simulink model "Spacecraft_Model_HAVOC"  (R2022b)
settings: Solver=VariableStepAuto  StartTime=0.0  StopTime=300  RelTol=1e-3
model workspace (MAT data in the model file):
  R_0 = 80000
  Ts = 0.01
  mu = 398600.435507
undefined symbols (not defined in the file): As, c, q, SC
libraries: simulink x6, cstblocks x6, aerolibnav x6, matrix_library x4, sharedtransform x4, sharedTrackingLibrary x3, aerolibgravity2 x3, aerolibutil x2, sharedutil x1
settings Model: Creator=rohin  LastModifiedBy=rohin

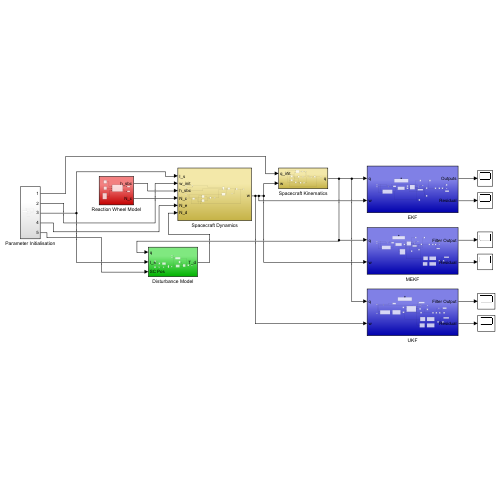
[thumbnail: Simulink's stored preview of the top-level diagram]
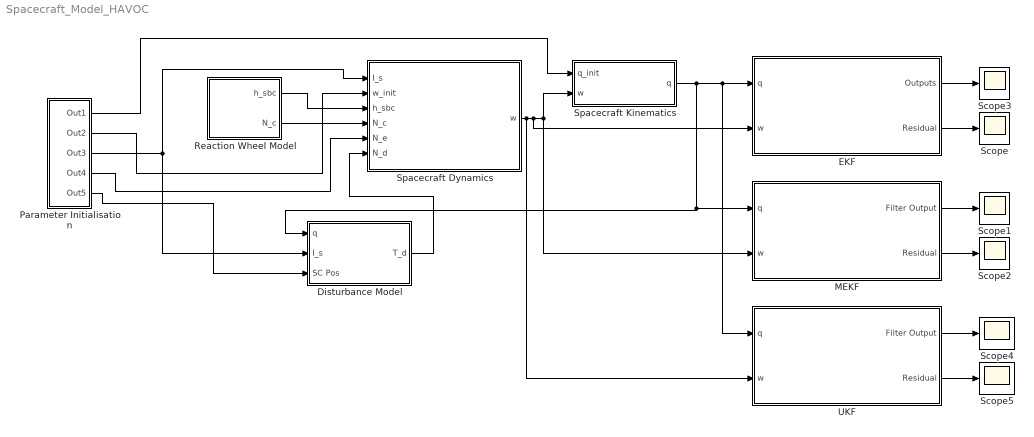
== system Spacecraft_Model_HAVOC ==
  Disturbance Model : Subsystem
  EKF : Subsystem
  MEKF : Subsystem
  Parameter Initialisation : Subsystem
  Reaction Wheel Model : Subsystem
  Scope{,1..5} (6 alike) : Scope
  Spacecraft Dynamics : Subsystem
  Spacecraft Kinematics : Subsystem
  UKF : Subsystem
  wires:
  Spacecraft Kinematics/1(q) -> MEKF/1(q), Disturbance Model/1(q), UKF/1(q), EKF/1(q)
  Spacecraft Dynamics/1(w) -> UKF/2(w), EKF/2(w), Spacecraft Kinematics/2(w), MEKF/2(w)
  EKF/1(Outputs) -> Scope3/1
  Reaction Wheel Model/1(h_sbc) -> Spacecraft Dynamics/3(h_sbc)
  Reaction Wheel Model/2(N_c) -> Spacecraft Dynamics/4(N_c)
  Disturbance Model/1(T_d) -> Spacecraft Dynamics/6(N_d)
  EKF/2(Residual) -> Scope/1
  MEKF/1(Filter Output) -> Scope1/1
  MEKF/2(Residual) -> Scope2/1
  UKF/1(Filter Output) -> Scope4/1
  UKF/2(Residual) -> Scope5/1
  Parameter Initialisation/3(Out3) -> Spacecraft Dynamics/1(I_s), Disturbance Model/2(I_s)
  Parameter Initialisation/1(Out1) -> Spacecraft Kinematics/1(q_init)
  Parameter Initialisation/2(Out2) -> Spacecraft Dynamics/2(w_init)
  Parameter Initialisation/4(Out4) -> Spacecraft Dynamics/5(N_e)
  Parameter Initialisation/5(Out5) -> Disturbance Model/3(SC Pos)

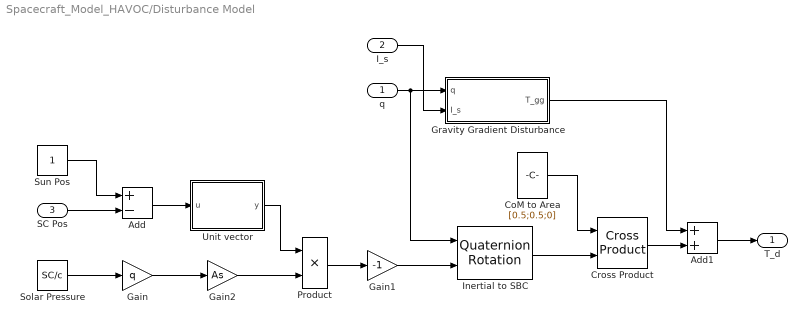
== system Spacecraft_Model_HAVOC/Disturbance Model ==
  q : Inport
  I_s : Inport  Port=2
  SC Pos : Inport  Port=3
  Add : Sum  Inputs=+-
  Add1 : Sum
  CoM to Area : Constant  Value=[0.5;0.5;0]  VectorParams1D=off
  Cross Product : matrix_library/Cross Product
  Gain : Gain  Gain=q
  Gain1 : Gain  Gain=-1
  Gain2 : Gain  Gain=As
  Gravity Gradient Disturbance : Subsystem
  Inertial to SBC : aerolibutil/Quaternion Rotation
  Product : Product
  Solar Pressure : Constant  Value=SC/c
  Sun Pos : Constant
  Unit vector : MATLAB Function  TreatAsAtomicUnit=on
  T_d : Outport
  wires:
  Sun Pos/1 -> Add/1
  Solar Pressure/1 -> Gain/1
  Unit vector/1(y) -> Product/1
  q/1 -> Gravity Gradient Disturbance/1(q), Inertial to SBC/1
  SC Pos/1 -> Add/2
  Add/1 -> Unit vector/1(u)
  I_s/1 -> Gravity Gradient Disturbance/2(I_s)
  Gain/1 -> Gain2/1
  Gain2/1 -> Product/2
  Product/1 -> Gain1/1
  Gain1/1 -> Inertial to SBC/2
  Gravity Gradient Disturbance/1(T_gg) -> Add1/1
  CoM to Area/1 -> Cross Product/1
  Inertial to SBC/1 -> Cross Product/2
  Cross Product/1 -> Add1/2
  Add1/1 -> T_d/1

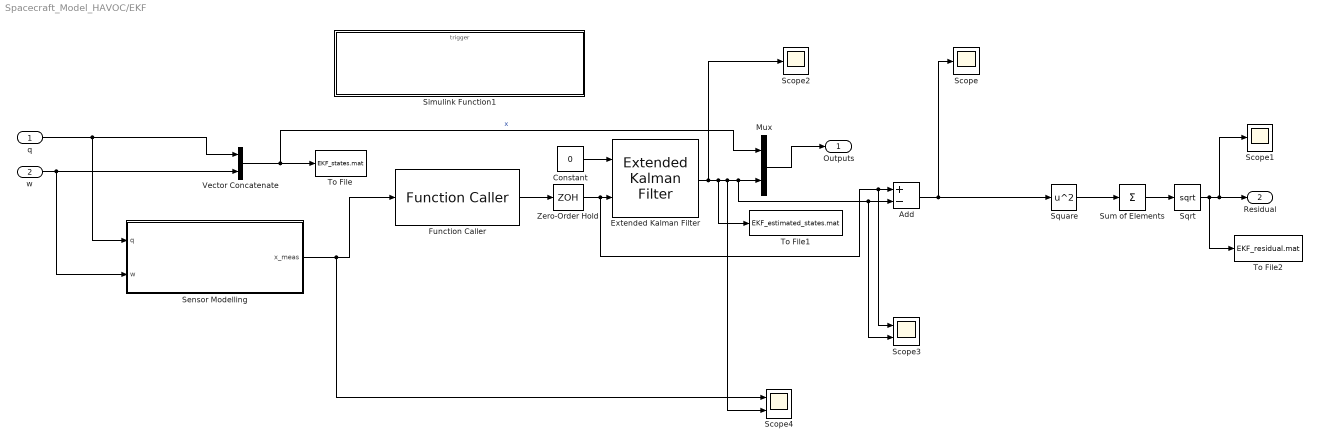
== system Spacecraft_Model_HAVOC/EKF ==
  q : Inport
  w : Inport  Port=2
  Add : Sum  Inputs=+-
  Constant : Constant  Value=0
  Extended Kalman Filter : sharedTrackingLibrary/Extended Kalman Filter  StateTransitionFcn=EKF_state_transition_func  HasStateTransitionJacobianFcn=off  HasAdditiveProcessNoise=Additive  ProcessNoise=0.05*diag([1,1,1,1,1,1,1])  HasTimeVaryingProcessNoise=off  HasStateTransitionFcnExtraArgument=1  InitialState=[1;0;0;0;0;0;0]  InitialStateCovariance=1  MeasurementFcn1=sensorMeasurementFcn  HasMeasurementJacobianFcn1=off  HasMeasurementEnablePort1=off  HasAdditiveMeasurementNoise1=Additive  MeasurementNoise1=0.1^2*diag([1,1,1,1,1,1,1])  HasTimeVaryingMeasurementNoise1=off  HasMeasurementFcnExtraArgument1=0  HasMeasurementWrapping1=off  MeasurementFcn2=myMeasurementFcn  HasMeasurementJacobianFcn2=off  HasMeasurementEnablePort2=off  HasAdditiveMeasurementNoise2=Additive  MeasurementNoise2=1  HasTimeVaryingMeasurementNoise2=off  HasMeasurementFcnExtraArgument2=0  HasMeasurementWrapping2=off  MeasurementFcn3=myMeasurementFcn  HasMeasurementJacobianFcn3=off  HasMeasurementEnablePort3=off  HasAdditiveMeasurementNoise3=Additive  MeasurementNoise3=1  HasTimeVaryingMeasurementNoise3=off  HasMeasurementFcnExtraArgument3=0  HasMeasurementWrapping3=off  MeasurementFcn4=myMeasurementFcn  HasMeasurementJacobianFcn4=off  HasMeasurementEnablePort4=off  HasAdditiveMeasurementNoise4=Additive  MeasurementNoise4=1  HasTimeVaryingMeasurementNoise4=off  HasMeasurementFcnExtraArgument4=0  HasMeasurementWrapping4=off  MeasurementFcn5=myMeasurementFcn  HasMeasurementJacobianFcn5=off  HasMeasurementEnablePort5=off  HasAdditiveMeasurementNoise5=Additive  MeasurementNoise5=1  HasTimeVaryingMeasurementNoise5=off  HasMeasurementFcnExtraArgument5=0  HasMeasurementWrapping5=off  EnableMultirate=off  StateTransitionFcnSampleTime=1  MeasurementFcn1SampleTime=1  MeasurementFcn2SampleTime=1  MeasurementFcn3SampleTime=1  MeasurementFcn4SampleTime=1  MeasurementFcn5SampleTime=1  UseCurrentEstimator=on  OutputStateCovariance=off  DataType=double  SampleTime=0.01  NumberOfMeasurements=1
  Function Caller : FunctionCaller  FunctionPrototype=y = sensorMeasurementFcn(x)  InputArgumentSpecifications=<Enter example>  OutputArgumentSpecifications=<Enter example>
  Mux : Mux  Inputs=2
  Scope : Scope
  Scope1 : Scope
  Scope2 : Scope
  Scope3 : Scope  NumInputPorts=2
  Scope4 : Scope  NumInputPorts=2
  "Sensor Modelling " : Subsystem
  Simulink Function1 : Subsystem  TreatAsAtomicUnit=on
  Sqrt : Sqrt
  Square : Math  Operator=square
  Sum of Elements : Sum  Inputs=+
  To File : ToFile  Filename=EKF_states.mat
  To File1 : ToFile  Filename=EKF_estimated_states.mat
  To File2 : ToFile  Filename=EKF_residual.mat
  Vector Concatenate : Concatenate
  Zero-Order Hold : ZeroOrderHold  SampleTime=0.01
  Outputs : Outport
  Residual : Outport  Port=2
  wires:
  Constant/1 -> Extended Kalman Filter/1
  w/1 -> "Sensor Modelling "/2(w), Vector Concatenate/2
  q/1 -> "Sensor Modelling "/1(q), Vector Concatenate/1
  Vector Concatenate/1 -> Mux/1, To File/1  "x"
  Function Caller/1 -> Zero-Order Hold/1
  Mux/1 -> Outputs/1
  Add/1 -> Square/1, Scope/1
  Sqrt/1 -> To File2/1, Scope1/1, Residual/1
  Square/1 -> Sum of Elements/1
  Sum of Elements/1 -> Sqrt/1
  "Sensor Modelling "/1(x_meas) -> Scope4/1, Function Caller/1
  Zero-Order Hold/1 -> Scope3/1, Add/1, Extended Kalman Filter/2
  Extended Kalman Filter/1 -> Scope2/1, Scope4/2, Add/2, Scope3/2, Mux/2, To File1/1

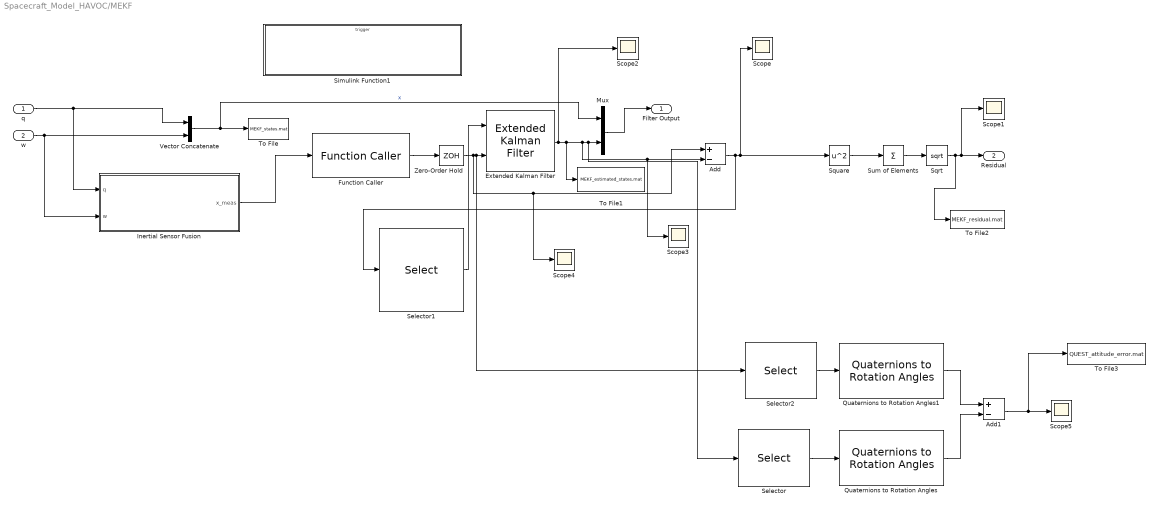
== system Spacecraft_Model_HAVOC/MEKF ==
  q : Inport
  w : Inport  Port=2
  Add : Sum  Inputs=+-
  Add1 : Sum  Inputs=+-
  Extended Kalman Filter : sharedTrackingLibrary/Extended Kalman Filter  StateTransitionFcn=MEKF_state_transition_func  HasStateTransitionJacobianFcn=off  HasAdditiveProcessNoise=Additive  ProcessNoise=0.5^2*diag([1,1,1,1,1,1,1])  HasTimeVaryingProcessNoise=off  HasStateTransitionFcnExtraArgument=1  InitialState=[1;0;0;0;0;0;0]  InitialStateCovariance=1  MeasurementFcn1=sensorMeasurementFcn  HasMeasurementJacobianFcn1=off  HasMeasurementEnablePort1=off  HasAdditiveMeasurementNoise1=Additive  MeasurementNoise1=0.01^2*diag([1,1,1,1,1,1,1])  HasTimeVaryingMeasurementNoise1=off  HasMeasurementFcnExtraArgument1=0  HasMeasurementWrapping1=off  MeasurementFcn2=myMeasurementFcn  HasMeasurementJacobianFcn2=off  HasMeasurementEnablePort2=off  HasAdditiveMeasurementNoise2=Additive  MeasurementNoise2=1  HasTimeVaryingMeasurementNoise2=off  HasMeasurementFcnExtraArgument2=0  HasMeasurementWrapping2=off  MeasurementFcn3=myMeasurementFcn  HasMeasurementJacobianFcn3=off  HasMeasurementEnablePort3=off  HasAdditiveMeasurementNoise3=Additive  MeasurementNoise3=1  HasTimeVaryingMeasurementNoise3=off  HasMeasurementFcnExtraArgument3=0  HasMeasurementWrapping3=off  MeasurementFcn4=myMeasurementFcn  HasMeasurementJacobianFcn4=off  HasMeasurementEnablePort4=off  HasAdditiveMeasurementNoise4=Additive  MeasurementNoise4=1  HasTimeVaryingMeasurementNoise4=off  HasMeasurementFcnExtraArgument4=0  HasMeasurementWrapping4=off  MeasurementFcn5=myMeasurementFcn  HasMeasurementJacobianFcn5=off  HasMeasurementEnablePort5=off  HasAdditiveMeasurementNoise5=Additive  MeasurementNoise5=1  HasTimeVaryingMeasurementNoise5=off  HasMeasurementFcnExtraArgument5=0  HasMeasurementWrapping5=off  EnableMultirate=off  StateTransitionFcnSampleTime=1  MeasurementFcn1SampleTime=1  MeasurementFcn2SampleTime=1  MeasurementFcn3SampleTime=1  MeasurementFcn4SampleTime=1  MeasurementFcn5SampleTime=1  UseCurrentEstimator=on  OutputStateCovariance=off  DataType=double  SampleTime=0.01  NumberOfMeasurements=1
  Function Caller : FunctionCaller  FunctionPrototype=y = sensorMeasurementFcn(x)  InputArgumentSpecifications=<Enter example>  OutputArgumentSpecifications=<Enter example>
  "Inertial Sensor Fusion " : Subsystem
  Mux : Mux  Inputs=2
  Quaternions to Rotation Angles : sharedtransform/Quaternions to Rotation Angles  rotationOrder=ZYX  aMode=aMode
  Quaternions to Rotation Angles1 : sharedtransform/Quaternions to Rotation Angles  rotationOrder=ZYX  aMode=aMode
  Scope{,1..5} (6 alike) : Scope
  Selector : Selector  InputPortWidth=7  IndexOptions=Index vector (dialog)  Indices=[1 2 3 4]  OutputSizes=1
  Selector1 : Selector  InputPortWidth=7  IndexOptions=Index vector (dialog)  Indices=[1 2 3 4]  OutputSizes=1
  Selector2 : Selector  InputPortWidth=7  IndexOptions=Index vector (dialog)  Indices=[1 2 3 4]  OutputSizes=1
  Simulink Function1 : Subsystem  TreatAsAtomicUnit=on
  Sqrt : Sqrt
  Square : Math  Operator=square
  Sum of Elements : Sum  Inputs=+
  To File : ToFile  Filename=MEKF_states.mat
  To File1 : ToFile  Filename=MEKF_estimated_states.mat
  To File2 : ToFile  Filename=MEKF_residual.mat
  To File3 : ToFile  Filename=QUEST_attitude_error.mat
  Vector Concatenate : Concatenate
  Zero-Order Hold : ZeroOrderHold  SampleTime=0.01
  Filter Output : Outport
  Residual : Outport  Port=2
  wires:
  Selector1/1 -> Extended Kalman Filter/1
  w/1 -> "Inertial Sensor Fusion "/2(w), Vector Concatenate/2
  q/1 -> "Inertial Sensor Fusion "/1(q), Vector Concatenate/1
  Vector Concatenate/1 -> Mux/1, To File/1  "x"
  Function Caller/1 -> Zero-Order Hold/1
  Mux/1 -> Filter Output/1
  "Inertial Sensor Fusion "/1(x_meas) -> Function Caller/1
  Sqrt/1 -> To File2/1, Scope1/1, Residual/1
  Square/1 -> Sum of Elements/1
  Sum of Elements/1 -> Sqrt/1
  Add/1 -> Selector1/1, Square/1, Scope/1
  Quaternions to Rotation Angles/1 -> Add1/2
  Quaternions to Rotation Angles1/1 -> Add1/1
  Add1/1 -> To File3/1, Scope5/1
  Zero-Order Hold/1 -> Scope4/1, Add/1, Selector2/1, Extended Kalman Filter/2
  Selector2/1 -> Quaternions to Rotation Angles1/1
  Selector/1 -> Quaternions to Rotation Angles/1
  Extended Kalman Filter/1 -> Scope2/1, Scope3/1, Add/2, Selector/1, Mux/2, To File1/1

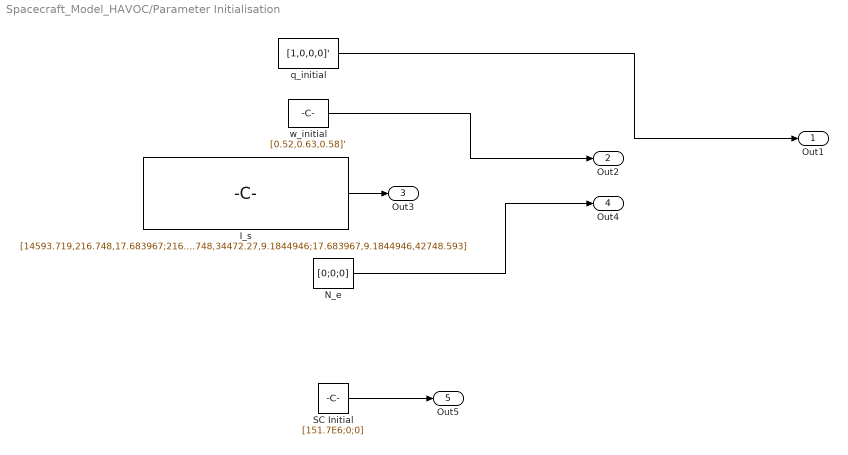
== system Spacecraft_Model_HAVOC/Parameter Initialisation ==
  I_s : Constant  Value=[14593.719,216.748,17.683967;216.748,34472.27,9.1844946;17.683967,9.1844946,42748.593]  VectorParams1D=off
  N_e : Constant  Value=[0;0;0]  VectorParams1D=off
  SC Initial : Constant  Value=[151.7E6;0;0]  VectorParams1D=off
  q_initial : Constant  Value=[1,0,0,0]'
  w_initial : Constant  Value=[0.52,0.63,0.58]'  VectorParams1D=off
  Out1 : Outport
  Out2 : Outport  Port=2
  Out3 : Outport  Port=3
  Out4 : Outport  Port=4
  Out5 : Outport  Port=5
  wires:
  I_s/1 -> Out3/1
  q_initial/1 -> Out1/1
  N_e/1 -> Out4/1
  w_initial/1 -> Out2/1
  SC Initial/1 -> Out5/1

== system Spacecraft_Model_HAVOC/Reaction Wheel Model ==
  N_d : Constant  Value=[5;0;0;0]  VectorParams1D=off
  Reaction Wheels : Subsystem
  beta : Constant  Value=45
  theta : Constant  Value=45
  h_sbc : Outport
  N_c : Outport  Port=2
  wires:
  Reaction Wheels/1(N_c) -> N_c/1
  beta/1 -> Reaction Wheels/2(beta)
  theta/1 -> Reaction Wheels/1(theta)
  N_d/1 -> Reaction Wheels/3(N_d)
  Reaction Wheels/2(h_sbc) -> h_sbc/1

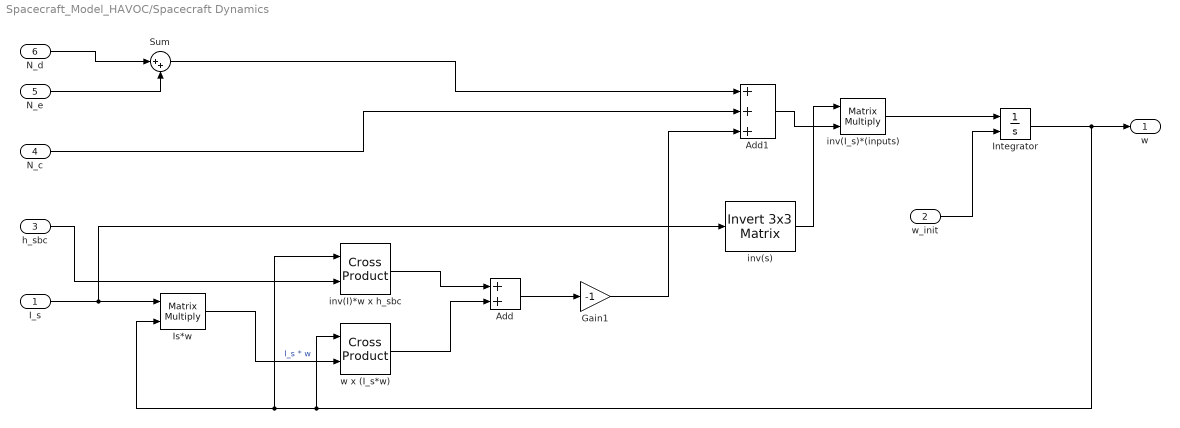
== system Spacecraft_Model_HAVOC/Spacecraft Dynamics ==
  I_s : Inport
  w_init : Inport  Port=2
  h_sbc : Inport  Port=3
  N_c : Inport  Port=4
  N_e : Inport  Port=5
  N_d : Inport  Port=6
  Add : Sum
  Add1 : Sum  Inputs=+++
  Gain1 : Gain  Gain=-1
  Integrator : Integrator  InitialConditionSource=external
  Is*w : Product  Multiplication=Matrix(*)
  Sum : Sum  Inputs=|++
  inv(I)*w x h_sbc : matrix_library/Cross Product
  inv(I_s)*(inputs) : Product  Multiplication=Matrix(*)
  inv(s) : aerolibutil/Invert  3x3 Matrix
  w x (I_s*w) : matrix_library/Cross Product
  w : Outport
  wires:
  w_init/1 -> Integrator/2
  Is*w/1 -> w x (I_s*w)/2  "I_s * w"
  N_c/1 -> Add1/2
  inv(I_s)*(inputs)/1 -> Integrator/1
  Integrator/1 -> w x (I_s*w)/1, inv(I)*w x h_sbc/1, Is*w/2, w/1
  I_s/1 -> inv(s)/1, Is*w/1
  inv(s)/1 -> inv(I_s)*(inputs)/1
  Add1/1 -> inv(I_s)*(inputs)/2
  h_sbc/1 -> inv(I)*w x h_sbc/2
  N_e/1 -> Sum/2
  N_d/1 -> Sum/1
  Sum/1 -> Add1/1
  w x (I_s*w)/1 -> Add/2
  inv(I)*w x h_sbc/1 -> Add/1
  Add/1 -> Gain1/1
  Gain1/1 -> Add1/3

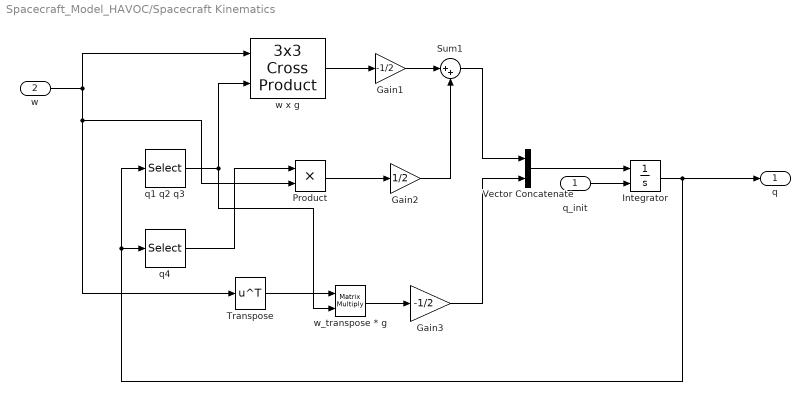
== system Spacecraft_Model_HAVOC/Spacecraft Kinematics ==
  q_init : Inport
  w : Inport  Port=2
  Gain1 : Gain  Gain=-1/2
  Gain2 : Gain  Gain=1/2
  Gain3 : Gain  Gain=-1/2
  Integrator : Integrator  InitialConditionSource=external
  Product : Product
  Sum1 : Sum  Inputs=|++
  Transpose : Math  Operator=transpose
  Vector Concatenate : Concatenate
  q1 q2 q3 : Selector  InputPortWidth=4  IndexOptions=Index vector (dialog)  Indices=[1 2 3]  OutputSizes=1
  q4 : Selector  InputPortWidth=4  IndexOptions=Index vector (dialog)  Indices=[4]  OutputSizes=1
  w x g : sharedutil/3x3 Cross Product  aMode=aMode
  w_transpose * g : Product  Multiplication=Matrix(*)
  q : Outport
  wires:
  Sum1/1 -> Vector Concatenate/1
  w_transpose * g/1 -> Gain3/1
  Gain1/1 -> Sum1/1
  Gain3/1 -> Vector Concatenate/2
  w x g/1 -> Gain1/1
  Gain2/1 -> Sum1/2
  w/1 -> Product/2, Transpose/1, w x g/1
  Transpose/1 -> w_transpose * g/1
  q1 q2 q3/1 -> w x g/2, w_transpose * g/2
  Vector Concatenate/1 -> Integrator/1
  q_init/1 -> Integrator/2
  Integrator/1 -> q/1, q1 q2 q3/1, q4/1
  q4/1 -> Product/1
  Product/1 -> Gain2/1

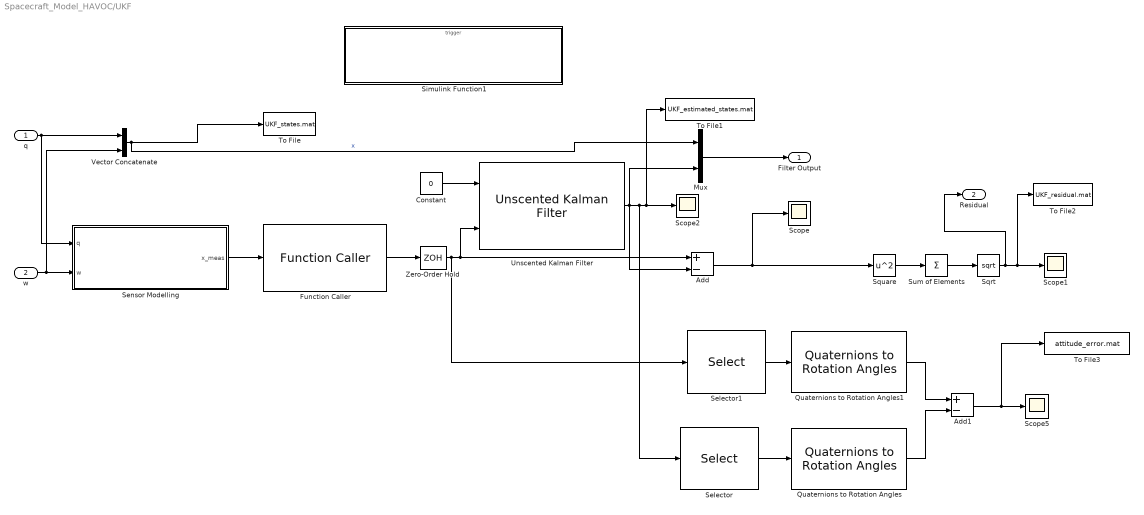
== system Spacecraft_Model_HAVOC/UKF ==
  q : Inport
  w : Inport  Port=2
  Add : Sum  Inputs=+-
  Add1 : Sum  Inputs=+-
  Constant : Constant  Value=0
  Function Caller : FunctionCaller  FunctionPrototype=y = UKF_sensorMeasurementFcn(x)  InputArgumentSpecifications=<Enter example>  OutputArgumentSpecifications=<Enter example>
  Mux : Mux  Inputs=2
  Quaternions to Rotation Angles : sharedtransform/Quaternions to Rotation Angles  rotationOrder=ZYX  aMode=aMode
  Quaternions to Rotation Angles1 : sharedtransform/Quaternions to Rotation Angles  rotationOrder=ZYX  aMode=aMode
  Scope{,1..2,5} (4 alike) : Scope
  Selector : Selector  InputPortWidth=7  IndexOptions=Index vector (dialog)  Indices=[1 2 3 4]  OutputSizes=1
  Selector1 : Selector  InputPortWidth=7  IndexOptions=Index vector (dialog)  Indices=[1 2 3 4]  OutputSizes=1
  "Sensor Modelling " : Subsystem
  Simulink Function1 : Subsystem  TreatAsAtomicUnit=on
  Sqrt : Sqrt
  Square : Math  Operator=square
  Sum of Elements : Sum  Inputs=+
  To File : ToFile  Filename=UKF_states.mat
  To File1 : ToFile  Filename=UKF_estimated_states.mat
  To File2 : ToFile  Filename=UKF_residual.mat
  To File3 : ToFile  Filename=attitude_error.mat
  Unscented Kalman Filter : sharedTrackingLibrary/Unscented Kalman Filter  StateTransitionFcn=UKF_state_transition_func  HasAdditiveProcessNoise=Additive  ProcessNoise=(0.1^2) * diag([0.01, 0.01, 0.01, 0.01, 0.01, 0.01, 0.01])  HasTimeVaryingProcessNoise=off  HasStateTransitionFcnExtraArgument=1  InitialState=[1;0;0;0;0;0;0]  InitialStateCovariance=0.01 * diag([0.01, 0.01, 0.01, 0.01, 0.01, 0.01, 0.01])  Alpha=1e-3  Beta=2  Kappa=0  MeasurementFcn1=UKF_sensorMeasurementFcn  HasMeasurementEnablePort1=off  HasAdditiveMeasurementNoise1=Additive  MeasurementNoise1=(0.001^2) * diag([0.01, 0.01, 0.01, 0.01, 0.01, 0.01, 0.01])  HasTimeVaryingMeasurementNoise1=off  HasMeasurementFcnExtraArgument1=0  HasMeasurementWrapping1=off  MeasurementFcn2=myMeasurementFcn  HasMeasurementEnablePort2=off  HasAdditiveMeasurementNoise2=Additive  MeasurementNoise2=1  HasTimeVaryingMeasurementNoise2=off  HasMeasurementFcnExtraArgument2=0  HasMeasurementWrapping2=off  MeasurementFcn3=myMeasurementFcn  HasMeasurementEnablePort3=off  HasAdditiveMeasurementNoise3=Additive  MeasurementNoise3=1  HasTimeVaryingMeasurementNoise3=off  HasMeasurementFcnExtraArgument3=0  HasMeasurementWrapping3=off  MeasurementFcn4=myMeasurementFcn  HasMeasurementEnablePort4=off  HasAdditiveMeasurementNoise4=Additive  MeasurementNoise4=1  HasTimeVaryingMeasurementNoise4=off  HasMeasurementFcnExtraArgument4=0  HasMeasurementWrapping4=off  MeasurementFcn5=myMeasurementFcn  HasMeasurementEnablePort5=off  HasAdditiveMeasurementNoise5=Additive  MeasurementNoise5=1  HasTimeVaryingMeasurementNoise5=off  HasMeasurementFcnExtraArgument5=0  HasMeasurementWrapping5=off  EnableMultirate=off  StateTransitionFcnSampleTime=1  MeasurementFcn1SampleTime=1  MeasurementFcn2SampleTime=1  MeasurementFcn3SampleTime=1  MeasurementFcn4SampleTime=1  MeasurementFcn5SampleTime=1  UseCurrentEstimator=on  OutputStateCovariance=off  DataType=double  SampleTime=0.01  NumberOfMeasurements=1
      settings: LibrarySourceBlock=cstblocks/State Estimation/Unscented Kalman Filter
  Vector Concatenate : Concatenate
  Zero-Order Hold : ZeroOrderHold  SampleTime=0.01
  Filter Output : Outport
  Residual : Outport  Port=2
  wires:
  q/1 -> "Sensor Modelling "/1(q), Vector Concatenate/1
  w/1 -> "Sensor Modelling "/2(w), Vector Concatenate/2
  Vector Concatenate/1 -> To File/1, Mux/1  "x"
  "Sensor Modelling "/1(x_meas) -> Function Caller/1
  Function Caller/1 -> Zero-Order Hold/1
  Constant/1 -> Unscented Kalman Filter/1
  Mux/1 -> Filter Output/1
  Add/1 -> Square/1, Scope/1
  Square/1 -> Sum of Elements/1
  Sum of Elements/1 -> Sqrt/1
  Sqrt/1 -> To File2/1, Scope1/1, Residual/1
  Quaternions to Rotation Angles/1 -> Add1/2
  Selector1/1 -> Quaternions to Rotation Angles1/1
  Quaternions to Rotation Angles1/1 -> Add1/1
  Unscented Kalman Filter/1 -> Selector/1, To File1/1, Scope2/1, Mux/2, Add/2
  Selector/1 -> Quaternions to Rotation Angles/1
  Zero-Order Hold/1 -> Selector1/1, Unscented Kalman Filter/2, Add/1
  Add1/1 -> To File3/1, Scope5/1

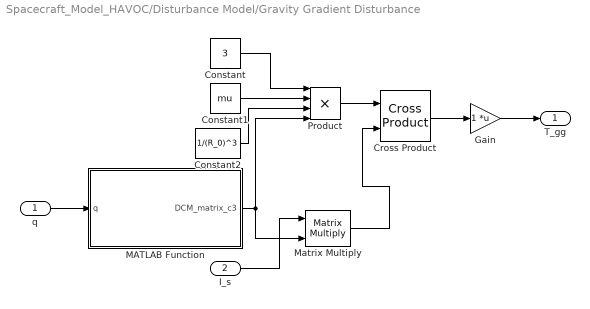
== system Spacecraft_Model_HAVOC/Disturbance Model/Gravity Gradient Disturbance ==
  q : Inport
  I_s : Inport  Port=2
  Constant : Constant  Value=3
  Constant1 : Constant  Value=mu
  Constant2 : Constant  Value=1/(R_0)^3
  Cross Product : matrix_library/Cross Product
  Gain : Gain  Multiplication=Matrix(K*u)
  MATLAB Function : MATLAB Function  TreatAsAtomicUnit=on
  Matrix Multiply : Product  Multiplication=Matrix(*)
  Product : Product  Inputs=4
  T_gg : Outport
  wires:
  q/1 -> MATLAB Function/1(q)
  Constant/1 -> Product/1
  Product/1 -> Cross Product/1
  MATLAB Function/1(DCM_matrix_c3) -> Matrix Multiply/2, Product/4
  Constant1/1 -> Product/2
  I_s/1 -> Matrix Multiply/1
  Matrix Multiply/1 -> Cross Product/2
  Constant2/1 -> Product/3
  Cross Product/1 -> Gain/1
  Gain/1 -> T_gg/1

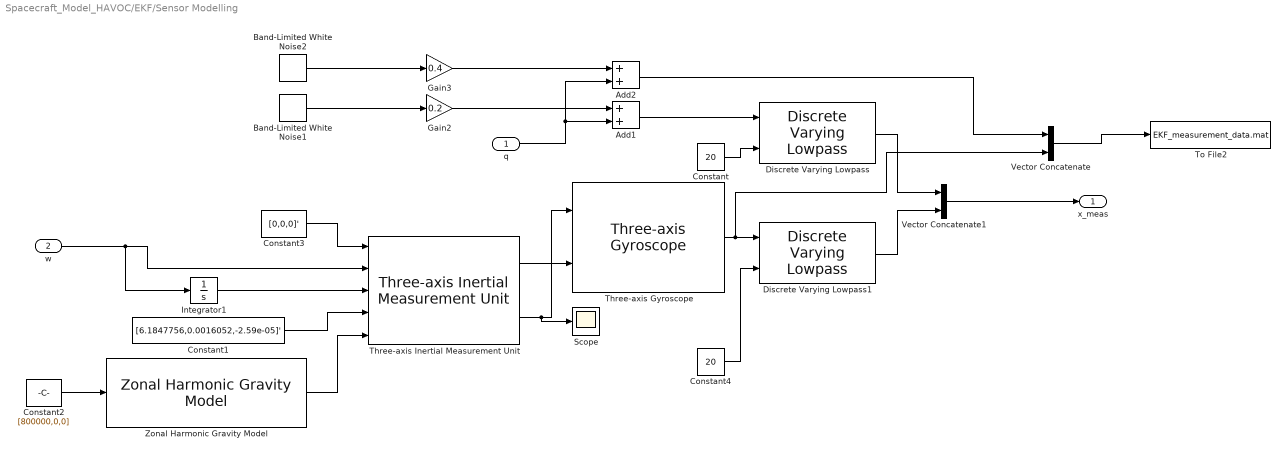
== system Spacecraft_Model_HAVOC/EKF/Sensor Modelling  ==
  q : Inport
  w : Inport  Port=2
  Add1 : Sum
  Add2 : Sum
  Band-Limited White Noise1 : simulink/Sources/Band-Limited White Noise  Cov=0.01  Ts=0.1  seed=[23341]
  Band-Limited White Noise2 : simulink/Sources/Band-Limited White Noise  Cov=0.01  Ts=0.1  seed=[23145]
  Constant : Constant  Value=20
  Constant1 : Constant  Value=[6.1847756,0.0016052,-2.59e-05]'
  Constant2 : Constant  Value=[800000,0,0]
  Constant3 : Constant  Value=[0,0,0]'
  Constant4 : Constant  Value=20
  Discrete Varying Lowpass : cstblocks/Linear Parameter Varying/Discrete Varying Lowpass  N=2  w0=0  Ts=0.01
  Discrete Varying Lowpass1 : cstblocks/Linear Parameter Varying/Discrete Varying Lowpass  N=2  w0=0  Ts=0.01
  Gain2 : Gain  Gain=0.2
  Gain3 : Gain  Gain=0.4
  Integrator1 : Integrator
  Scope : Scope
  Three-axis Gyroscope : aerolibnav/Three-axis Gyroscope  dtype_g=on  w_g=190  z_g=0.707  g_sf_cc=[1 0 0; 0 1 0; 0 0 1]  g_bias=0.0005*[1 1 1]  g_sen=[0 0 0]  g_Ts=0  g_rand=on  g_seeds=[23093 23094 23095]  g_pow=[0.0001 0.0001 0.0001]  g_sat="[-inf  -inf  -inf  inf inf inf]"
  Three-axis Inertial Measurement Unit : aerolibnav/Three-axis Inertial Measurement Unit  units=Metric (MKS)  imu=[0 0 0]  i_Ts=0  dtype_a=on  w_a=190  z_a=0.707  a_sf_cc=[1 0 0; 0 1 0; 0 0 1]  a_bias=[0 0 0]  a_sat="[-inf  -inf  -inf  inf inf inf]"  dtype_g=on  w_g=190  z_g=0.707  g_sf_cc=[1 0 0; 0 1 0; 0 0 1]  g_bias=[0 0 0]  g_sens=[0 0 0]  g_sat="[-inf  -inf  -inf  inf inf inf]"  i_rand=on  i_seeds=[23093 23094 23095 23096 23097 23098]  i_pow=[0.001 0.001 0.001 0.0001 0.0001 0.0001]
  To File2 : ToFile  Filename=EKF_measurement_data.mat
  Vector Concatenate : Concatenate
  Vector Concatenate1 : Concatenate
  Zonal Harmonic Gravity Model : aerolibgravity2/Zonal Harmonic Gravity Model  units=Metric (MKS)  degree=4  action=Warning  ptype=Earth  R=6378136.3  GM=398600441500000  jvalue=[1.0826269e-03 -2.5323000e-06 -1.6204000e-06]
  x_meas : Outport
  wires:
  Gain3/1 -> Add2/1
  Constant3/1 -> Three-axis Inertial Measurement Unit/1
  w/1 -> Three-axis Inertial Measurement Unit/2, Integrator1/1
  Band-Limited White Noise2/1 -> Gain3/1
  Constant2/1 -> Zonal Harmonic Gravity Model/1
  Integrator1/1 -> Three-axis Inertial Measurement Unit/3
  Band-Limited White Noise1/1 -> Gain2/1
  Discrete Varying Lowpass1/1 -> Vector Concatenate1/2
  Constant1/1 -> Three-axis Inertial Measurement Unit/4
  Discrete Varying Lowpass/1 -> Vector Concatenate1/1
  Zonal Harmonic Gravity Model/1 -> Three-axis Inertial Measurement Unit/5
  Gain2/1 -> Add1/1
  q/1 -> Add2/2, Add1/2
  Add1/1 -> Discrete Varying Lowpass/1
  Three-axis Inertial Measurement Unit/2 -> Three-axis Gyroscope/1, Scope/1
  Three-axis Inertial Measurement Unit/1 -> Three-axis Gyroscope/2
  Add2/1 -> Vector Concatenate/1
  Constant/1 -> Discrete Varying Lowpass/2
  Three-axis Gyroscope/1 -> Vector Concatenate/2, Discrete Varying Lowpass1/1
  Constant4/1 -> Discrete Varying Lowpass1/2
  Vector Concatenate1/1 -> x_meas/1
  Vector Concatenate/1 -> To File2/1

== system Spacecraft_Model_HAVOC/EKF/Simulink Function1 ==
  sensorMeasurementFcn : TriggerPort  TriggerType=function-call  IsSimulinkFunction=on  FunctionName=sensorMeasurementFcn  FunctionVisibility=scoped  VariantControl=(inherit)
  x : ArgIn  DisableCoverage=on  PortDimensions=7  ArgumentName=x
  y : ArgOut  DisableCoverage=on  PortDimensions=7  ArgumentName=y
  wires:
  x/1 -> y/1

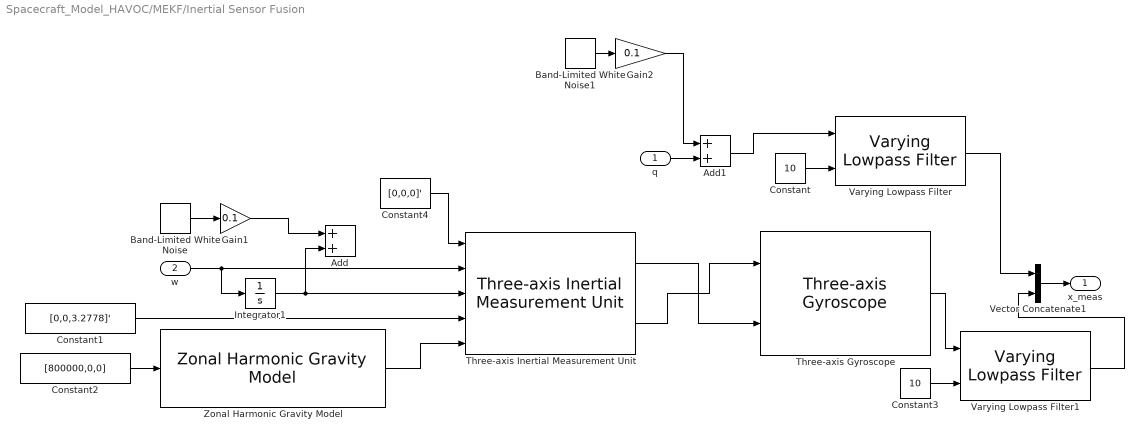
== system Spacecraft_Model_HAVOC/MEKF/Inertial Sensor Fusion  ==
  q : Inport
  w : Inport  Port=2
  Add : Sum
  Add1 : Sum
  Band-Limited White Noise : simulink/Sources/Band-Limited White Noise  Cov=[0.01]  Ts=0.1  seed=[26349]
  Band-Limited White Noise1 : simulink/Sources/Band-Limited White Noise  Cov=0.01  Ts=0.1  seed=[23741]
  Constant : Constant  Value=10
  Constant1 : Constant  Value=[0,0,3.2778]'
  Constant2 : Constant  Value=[800000,0,0]
  Constant3 : Constant  Value=10
  Constant4 : Constant  Value=[0,0,0]'
  Gain1 : Gain  Gain=0.1
  Gain2 : Gain  Gain=0.1
  Integrator1 : Integrator
  Three-axis Gyroscope : aerolibnav/Three-axis Gyroscope  dtype_g=on  w_g=190  z_g=0.707  g_sf_cc=[1 0 0; 0 1 0; 0 0 1]  g_bias=0.0005*[1 1 1]  g_sen=[0 0 0]  g_Ts=0  g_rand=on  g_seeds=[23093 23094 23095]  g_pow=[0.0001 0.0001 0.0001]  g_sat="[-inf  -inf  -inf  inf inf inf]"
  Three-axis Inertial Measurement Unit : aerolibnav/Three-axis Inertial Measurement Unit  units=Metric (MKS)  imu=[0 0 0]  i_Ts=0  dtype_a=on  w_a=190  z_a=0.707  a_sf_cc=[1 0 0; 0 1 0; 0 0 1]  a_bias=[0 0 0]  a_sat="[-inf  -inf  -inf  inf inf inf]"  dtype_g=on  w_g=190  z_g=0.707  g_sf_cc=[1 0 0; 0 1 0; 0 0 1]  g_bias=[0 0 0]  g_sens=[0 0 0]  g_sat="[-inf  -inf  -inf  inf inf inf]"  i_rand=on  i_seeds=[23093 23094 23095 23096 23097 23098]  i_pow=[0.001 0.001 0.001 0.0001 0.0001 0.0001]
  Varying Lowpass Filter : cstblocks/Linear Parameter Varying/Varying Lowpass Filter  N=1
  Varying Lowpass Filter1 : cstblocks/Linear Parameter Varying/Varying Lowpass Filter  N=1
  Vector Concatenate1 : Concatenate
  Zonal Harmonic Gravity Model : aerolibgravity2/Zonal Harmonic Gravity Model  units=Metric (MKS)  degree=4  action=Warning  ptype=Earth  R=6378136.3  GM=398600441500000  jvalue=[1.0826269e-03 -2.5323000e-06 -1.6204000e-06]
  x_meas : Outport
  wires:
  Three-axis Inertial Measurement Unit/2 -> Three-axis Gyroscope/1
  Integrator1/1 -> Add/2, Three-axis Inertial Measurement Unit/3
  Zonal Harmonic Gravity Model/1 -> Three-axis Inertial Measurement Unit/5
  Three-axis Inertial Measurement Unit/1 -> Three-axis Gyroscope/2
  w/1 -> Three-axis Inertial Measurement Unit/2, Integrator1/1
  Constant2/1 -> Zonal Harmonic Gravity Model/1
  Constant1/1 -> Three-axis Inertial Measurement Unit/4
  Band-Limited White Noise/1 -> Gain1/1
  Gain1/1 -> Add/1
  Band-Limited White Noise1/1 -> Gain2/1
  Gain2/1 -> Add1/1
  Vector Concatenate1/1 -> x_meas/1
  q/1 -> Add1/2
  Add1/1 -> Varying Lowpass Filter/1
  Constant/1 -> Varying Lowpass Filter/2
  Varying Lowpass Filter/1 -> Vector Concatenate1/1
  Three-axis Gyroscope/1 -> Varying Lowpass Filter1/1
  Varying Lowpass Filter1/1 -> Vector Concatenate1/2
  Constant3/1 -> Varying Lowpass Filter1/2
  Constant4/1 -> Three-axis Inertial Measurement Unit/1

== system Spacecraft_Model_HAVOC/MEKF/Simulink Function1 ==
  sensorMeasurementFcn : TriggerPort  TriggerType=function-call  IsSimulinkFunction=on  FunctionName=sensorMeasurementFcn  FunctionVisibility=scoped  VariantControl=(inherit)
  x : ArgIn  DisableCoverage=on  PortDimensions=7  ArgumentName=x
  y : ArgOut  DisableCoverage=on  PortDimensions=7  ArgumentName=y
  wires:
  x/1 -> y/1

== system Spacecraft_Model_HAVOC/Reaction Wheel Model/Reaction Wheels ==
  theta : Inport
  beta : Inport  Port=2
  N_d : Inport  Port=3
  Gain : Gain  Gain=-1
  Integrator : Integrator
  MATLAB Function1 : MATLAB Function  TreatAsAtomicUnit=on
  Matrix Multiply : Product  Multiplication=Matrix(*)
  Matrix Multiply1 : Product  Multiplication=Matrix(*)
  N_c : Outport
  h_sbc : Outport  Port=2
  wires:
  theta/1 -> MATLAB Function1/1(theta)
  beta/1 -> MATLAB Function1/2(beta)
  MATLAB Function1/1(A_w) -> Matrix Multiply1/1, Matrix Multiply/1
  N_d/1 -> Gain/1, Integrator/1
  Integrator/1 -> Matrix Multiply/2  "h_w"
  Gain/1 -> Matrix Multiply1/2
  Matrix Multiply1/1 -> N_c/1
  Matrix Multiply/1 -> h_sbc/1

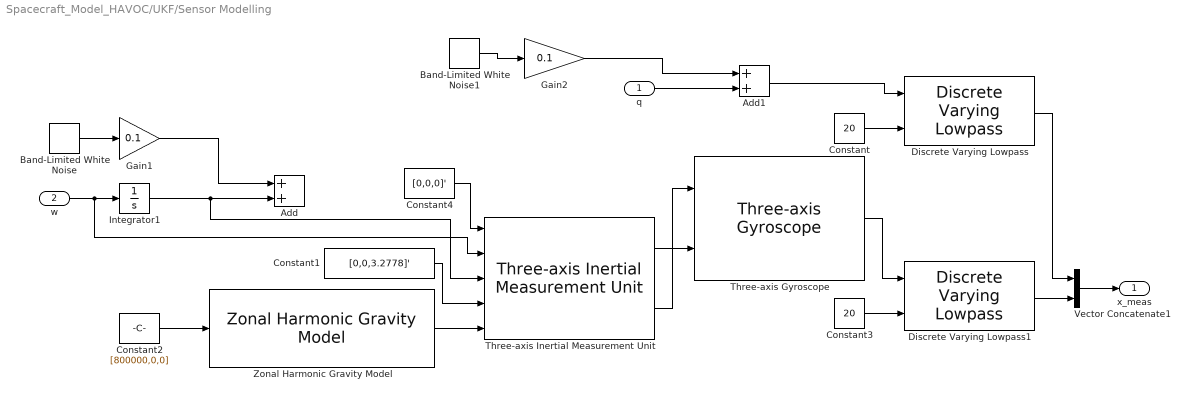
== system Spacecraft_Model_HAVOC/UKF/Sensor Modelling  ==
  q : Inport
  w : Inport  Port=2
  Add : Sum
  Add1 : Sum
  Band-Limited White Noise : simulink/Sources/Band-Limited White Noise  Cov=[0.01]  Ts=0.1  seed=[22391]
  Band-Limited White Noise1 : simulink/Sources/Band-Limited White Noise  Cov=0.01  Ts=0.1  seed=[27381]
  Constant : Constant  Value=20
  Constant1 : Constant  Value=[0,0,3.2778]'
  Constant2 : Constant  Value=[800000,0,0]
  Constant3 : Constant  Value=20
  Constant4 : Constant  Value=[0,0,0]'
  Discrete Varying Lowpass : cstblocks/Linear Parameter Varying/Discrete Varying Lowpass  N=2  w0=10  Ts=0.01
  Discrete Varying Lowpass1 : cstblocks/Linear Parameter Varying/Discrete Varying Lowpass  N=2  w0=10  Ts=0.01
  Gain1 : Gain  Gain=0.1
  Gain2 : Gain  Gain=0.1
  Integrator1 : Integrator
  Three-axis Gyroscope : aerolibnav/Three-axis Gyroscope  dtype_g=on  w_g=190  z_g=0.707  g_sf_cc=[1 0 0; 0 1 0; 0 0 1]  g_bias=0.0005*[1 1 1]  g_sen=[0 0 0]  g_Ts=0  g_rand=on  g_seeds=[23093 23094 23095]  g_pow=[0.0001 0.0001 0.0001]  g_sat="[-inf  -inf  -inf  inf inf inf]"
  Three-axis Inertial Measurement Unit : aerolibnav/Three-axis Inertial Measurement Unit  units=Metric (MKS)  imu=[0 0 0]  i_Ts=0  dtype_a=on  w_a=190  z_a=0.707  a_sf_cc=[1 0 0; 0 1 0; 0 0 1]  a_bias=[0 0 0]  a_sat="[-inf  -inf  -inf  inf inf inf]"  dtype_g=on  w_g=190  z_g=0.707  g_sf_cc=[1 0 0; 0 1 0; 0 0 1]  g_bias=[0 0 0]  g_sens=[0 0 0]  g_sat="[-inf  -inf  -inf  inf inf inf]"  i_rand=on  i_seeds=[23093 23094 23095 23096 23097 23098]  i_pow=[0.001 0.001 0.001 0.0001 0.0001 0.0001]
  Vector Concatenate1 : Concatenate
  Zonal Harmonic Gravity Model : aerolibgravity2/Zonal Harmonic Gravity Model  units=Metric (MKS)  degree=4  action=Warning  ptype=Earth  R=6378136.3  GM=398600441500000  jvalue=[1.0826269e-03 -2.5323000e-06 -1.6204000e-06]
  x_meas : Outport
  wires:
  Band-Limited White Noise1/1 -> Gain2/1
  Band-Limited White Noise/1 -> Gain1/1
  w/1 -> Integrator1/1, Three-axis Inertial Measurement Unit/2
  Constant2/1 -> Zonal Harmonic Gravity Model/1
  Gain1/1 -> Add/1
  Constant1/1 -> Three-axis Inertial Measurement Unit/4
  Integrator1/1 -> Three-axis Inertial Measurement Unit/3, Add/2
  Constant3/1 -> Discrete Varying Lowpass1/2
  Zonal Harmonic Gravity Model/1 -> Three-axis Inertial Measurement Unit/5
  Gain2/1 -> Add1/1
  q/1 -> Add1/2
  Three-axis Inertial Measurement Unit/1 -> Three-axis Gyroscope/2
  Discrete Varying Lowpass/1 -> Vector Concatenate1/1
  Three-axis Gyroscope/1 -> Discrete Varying Lowpass1/1
  Three-axis Inertial Measurement Unit/2 -> Three-axis Gyroscope/1
  Add1/1 -> Discrete Varying Lowpass/1
  Constant/1 -> Discrete Varying Lowpass/2
  Discrete Varying Lowpass1/1 -> Vector Concatenate1/2
  Vector Concatenate1/1 -> x_meas/1
  Constant4/1 -> Three-axis Inertial Measurement Unit/1

== system Spacecraft_Model_HAVOC/UKF/Simulink Function1 ==
  UKF_sensorMeasurementFcn : TriggerPort  TriggerType=function-call  IsSimulinkFunction=on  FunctionName=UKF_sensorMeasurementFcn  FunctionVisibility=scoped  VariantControl=(inherit)
  x : ArgIn  DisableCoverage=on  PortDimensions=7  ArgumentName=x
  y : ArgOut  DisableCoverage=on  PortDimensions=7  ArgumentName=y
  wires:
  x/1 -> y/1

== matlab function Spacecraft_Model_HAVOC/Disturbance Model/Gravity Gradient Disturbance/MATLAB Function ==
  data: q input; DCM_matrix_c3 output
function DCM_matrix_c3 = DCM(q)
    
    % Define the allocation matrix
    DCM_matrix = [(1 -2*(q(2)^2+q(3)^2)), 2*(q(1)*q(2) + q(3)*q(4)), 2*(q(1)*q(3) - q(2)*q(4));
        (2*(q(2)*q(1) - q(3)*q(4))), (1-2*(q(1)^2+q(3)^2)), (2*(q(2)*q(3) + q(1)*q(4)));
        (2*(q(3)*q(1) + q(2)*q(4))), (2*(q(3)*q(2)-q(1)*q(4))), (1-2*(q(1)^2+q(2)^2))];

    DCM_matrix_c3 = DCM_matrix(:,3);
end

== matlab function Spacecraft_Model_HAVOC/Disturbance Model/Unit vector ==
  data: u input; y output
function y = fcn(u)
y = u./norm(u);

== matlab function Spacecraft_Model_HAVOC/Reaction Wheel Model/Reaction Wheels/MATLAB Function1 ==
  data: theta input; A_w output; beta input
function A_w = reactionWheelAllocationMatrix(theta, beta)
    % Convert angles to radians
    theta = deg2rad(theta);
    beta = deg2rad(beta);
    
    % Define the allocation matrix
    A_w = [cos(beta)*cos(theta), -cos(beta)*sin(theta), -cos(beta)*cos(theta), cos(beta)*sin(theta);
           cos(beta)*sin(theta), cos(beta)*cos(theta), -cos(beta)*sin(theta), -cos(beta)*cos(theta);
           sin(beta), sin(beta), sin(beta), sin(beta)];
end
